simulink library "commblkcod"  (Simulink 5.0)
undefined symbols (not defined in the file or in its folder): G, gfprimfd, H, k, m, n, p
libraries: commutil x28, dspmtrx2 x14, commblkcod x12, commsource x12
settings Model: Creator=mikem  LastModifiedBy=mmclerno

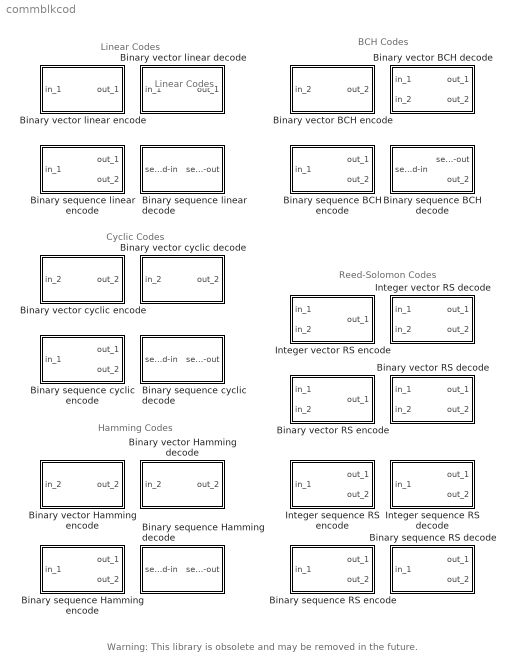
== system commblkcod ==
  note: Linear Codes
  note: Cyclic Codes
  note: Hamming Codes
  note: BCH Codes
  note: Reed-Solomon Codes
  note: Linear Codes
  note: Warning: This library is obsolete and may be removed in the future.
  Binary sequence BCH decode : Subsystem  mask(Sequence I/O BCH decode){n=15, k=5, t=3, samp=1/5}
      mask prompts: n "Codeword length N (N=2^M-1. M is a >2 integer):"; k "Message length K (check BCHPOLY for valid K):"; t "Error-correction capability T (0 for unknown):"; samp "Output sample time T_out (sec):"
      mask help: BCH decode with codeword length N, message length K, and error-correction capability T. (N,K,T) must be a valid BCH code combination.
      mask Help: This block decodes length N binary codeword into length K message using BCH code. The block uses sequential input/output format. The input sequence sample time is K*T_out/N. The block causes a K*T_out delay. The second outport outputs the number of errors detected in the process. A negative value indicates the block found more error in the codeword than T.
      mask Display: plot(0,0,100,100,[35 05 05 35 35 35 15 15 25 25 35 35 60 70 70 75 70 70 75 75 95 95 75 75 85 85],[95 95 85 85 95 85 85 95 95 85 85 90 90 90 93 90 87 93 90 95 95 85 85 95 95 85]-5);disp('BCH de')
  Binary sequence BCH encode : Subsystem  mask(Sequence I/O BCH encode){n=15, k=5, samp=1/5}
      mask prompts: n "Codeword length N (N=2^M-1. M is a >2 integer):"; k "Message length K (check BCHPOLY for valid K):"; samp "Input sample time T_in (sec):"
      mask help: BCH encode with codeword length N, and message length K. (N, K) must be a valid BCH code pair.
      mask init:
      | [x,y]=trigicon(1,75,get_param(gcb,'orientation'),1);
      mask Help: This block encodes length K binary message into length N binary codeword using BCH code. The block uses sequence input/output format. The output sequential sample time is K*T_in/N. The block causes a K*T_in delay. The second outport outputs a pulse when Kth message signal is received. Use function BCHPOLY to view the valid N, K, and error-corr ection capability T combination.
      mask Display: plot(0,0,100,100, [25 5 5 25 25 25 15 15 25 25 50 60 60 65 60 60 65 65 95 95 65 65 75 75 85 85],[90 90 80 80 90 80 80 90 90 85 85 85 88 85 82 88 85 90 90 80 80 90 90 80 80 90],x,y);disp('BCH en')
  Binary sequence Hamming decode : Subsystem  mask(Sequence I/O Hamming decode){n=7, k=gfprimfd(3,'min'), samp=1/4}
      mask prompts: n "Codeword length N:"; k "Message length K, or M-degree primitive polynomial:"; samp "Input sample time T_out (sec):"
      mask help: Single error-correction Hamming decode with codeword length N=2^M-1, message length K=2^M-M-1, where M is a >=3 integer.
      mask init:
      | if length(k)>1,p=k;k=n-length(p)+1;else,p=gfprimdf(n-k);end;
      mask Help: This block decodes length N binary codeword into length K message using Hamming code. The block uses sequential input/output format. The input sequence sample time is K*T_out/N. The block causes a K*T_out delay. Use function GFPRIMDF or GFPRIMFD to find M-degree\nprimitive polynomials.
      mask Display:
      | plot(0,0,100,100,[35 05 05 35 35 35 15 15 25 25 35 35 60 70 70 75 70 70 75 75 95 95 75 75 85 85],[95 95 85 85 95 85 85 95 95 85 85 90 90 90 93 90 87 93 90 95 95 85 85 95 95 85]-5);
      | disp('Hamming de')
  Binary sequence Hamming encode : Subsystem  mask(Sequence I/O Hamming encode){n=7, k=gfprimfd(3,'min'), samp=1/4}
      mask prompts: n "Codeword length N:"; k "Message length K, or M-degree primitive polynomial:"; samp "Input sample time T_in (sec):"
      mask help: Single error-correction Hamming encode with codeword length N=2^M-1, message length K=2^M-M-1, where M is a >=3 integer.
      mask init:
      | if length(k)>1,p=k;k=n-length(k)+1;else,p=gfprimdf(n-k);end;
      mask Help: This block encodes length K binary message into length N binary codeword using Hamming code. The block uses sequential input/output format. The output sequence sample time is K*T_in/N. The block causes a K*T_in delay. The second outport outputs a pulse when Kth message signal is received. Use function GFPRIMDF or GFPRIMFD to find M-degree\nprimitive polynomials.
      mask Display:
      | plot(0,0,100,100, [25 5 5 25 25 25 15 15 25 25 50 60 60 65 60 60 65 65 95 95 65 65 75 75 85 85],[90 90 80 80 90 80 80 90 90 85 85 85 88 85 82 88 85 90 90 80 80 90 90 80 80 90]);
      | disp('Hamming en')
  Binary sequence RS decode : Subsystem  mask(Binary sequence I/O RS decode){n=7, k=5, samp=1/5/3}
      mask prompts: n "Code length N=2^M-1 (M is a >2 integer):"; k "Message length K:"; samp "Output sample time T_out (sec):"
      mask help: RS decode with codeword length N, message length K.
      mask init:
      | m=3;p_d=7;while p_d<n,m=m+1;p_d=2^m-1;end;
      mask Help: This block decodes length N binary codeword into length K binary message. The block uses sequence input/output format. The input sequential sample time is K*T_out/N. The block causes a K*M*T_out delay. The second outport outputs the number of errors detected in the process. If the codeword contains more error than the correction capability, this output is nagative.
      mask Display:
      | plot(0,0,100,100,[35 05 05 35 35 35 15 15 25 25 35 35 60 70 70 75 70 70 75 75 95 95 75 75 85 85],[95 95 85 85 95 85 85 95 95 85 85 90 90 90 93 90 87 93 90 95 95 85 85 95 95 85]-5);
      | disp('B-RS de')
  Binary sequence RS encode : Subsystem  mask(Binary sequence I/O RS encode){n=7, k=5, samp=1/5/3}
      mask prompts: n "Code length N=2^M-1 (M is a >2 integer):"; k "Message length K:"; samp "Input sample time T_in (sec):"
      mask help: RS encode with codeword length N, message length K.
      mask init:
      | m=3;p_m=7;while p_m<n,m=m+1;p_m=2^m-1;end;
      mask Help: This block encodes length K binary message into length N binary codeword. The block uses sequential input/output format. The output sequence sample time is K*T_in/N. The block causes a K*M*T_in delay. The second outport outputs a pulse when (K*M)-th message signal is received.
      mask Display:
      | plot(0,0,100,100, [25 5 5 25 25 25 15 15 25 25 50 60 60 65 60 60 65 65 95 95 65 65 75 75 85 85],[90 90 80 80 90 80 80 90 90 85 85 85 88 85 82 88 85 90 90 80 80 90 90 80 80 90]);
      | disp('B-RS en')
  Binary sequence cyclic decode : Subsystem  mask(Sequence I/O cyclic decode){n=7, p=4, samp=1/4}
      mask prompts: n "Codeword length N:"; p "Message length K, or generator polynomial Pg:"; samp "Output sample time T_out (sec):"
      mask help: Sequence decode with codeword length N and message length K.
      mask init:
      | if length(p)==1, p=cyclpoly(n,p,'min');end;if isempty(p),error('No such cyclic code exist');end;k=n-length(p)+1;
      mask Help: This block decodes length N binary codeword into length K message using cyclic code. The block uses sequential input/output format. Use function CYCLPOLY for a list of cyclic generator polynomials. The input sequence sample time is K*T_out/N. The block causes a K*T_out delay.
      mask Display:
      | plot(0,0,100,100,[35 05 05 35 35 35 15 15 25 25 35 35 60 70 70 75 70 70 75 75 95 95 75 75 85 85],[95 95 85 85 95 85 85 95 95 85 85 90 90 90 93 90 87 93 90 95 95 85 85 95 95 85]-5);
      | disp('Cyclic de');
  Binary sequence cyclic encode : Subsystem  mask(Sequence I/O cyclic encode){n=7, p=4, samp=1/4}
      mask prompts: n "Codeword length N:"; p "Message length K, or generator polynomial Pg:"; samp "Input sample time T_in (sec):"
      mask help: Cyclic encode with codeword length N and message length K.
      mask init:
      | if length(p)==1,p=cyclpoly(n,p,'min');if isempty(p),error('No such cyclic code exist');end;end;k=n-length(p)+1;
      mask Help: This block encodes length K binary message into length N binary codeword using cyclic code. The block uses sequential input/output format. The output sequence sample time is K*T_in/N. The block causes a K*T_in delay. The second outport outputs a pulse when Kth message signal is received. Use function CYCLPOLY for a list of cyclic generator polynomials.
      mask Display:
      | plot(0,0,100,100, [25 5 5 25 25 25 15 15 25 25 50 60 60 65 60 60 65 65 95 95 65 65 75 75 85 85],[90 90 80 80 90 80 80 90 90 85 85 85 88 85 82 88 85 90 90 80 80 90 90 80 80 90]);
      | disp('Cyclic en')
  Binary sequence linear decode : Subsystem  mask(Sequence I/O linear block decode){G=[[1 1 0; 0 1 1; 1 1 1; 1 0 1] eye(4)], trt=0, samp=1/4}
      mask prompts: G "Generator matrix (binary K-by-N matrix):"; trt "Error-correction truth table (0 for single error-corr):"; samp "Output sample time T_out (sec):"
      mask help: Linear block decode with message length K and codeword length N.
      mask init:
      | [k,n]=size(G);
      mask Help: This block decodes length N binary codeword into length K message using linear block code. The block uses sequential input/output format. The input sequence sample time is K*T_out/N. The block causes a K*T_out delay. The generator matrix is a K-by-N matrix. Linear block code is a generic code.
      mask Display:
      | plot(0,0,100,100,[35 05 05 35 35 35 15 15 25 25 35 35 60 70 70 75 70 70 75 75 95 95 75 75 85 85],[95 95 85 85 95 85 85 95 95 85 85 90 90 90 93 90 87 93 90 95 95 85 85 95 95 85]-5);
      | disp('Linear de')
  Binary sequence linear encode : Subsystem  mask(Sequence I/O linear block encode){G=[[1 1 0; 0 1 1; 1 1 1; 1 0 1] eye(4)], samp=1/4}
      mask prompts: G "Generator matrix (binary K-by-N matrix):"; samp "Input sample time T_in (sec):"
      mask help: Linear block encode with message length K and codeword length N.
      mask init:
      | [k, n]=size(G);
      mask Help: This block encodes length K binary message into length N binary codeword using linear block code. The block uses sequential input/output format. The output sequence sample time is K*T_in/N. The block causes a K*T_in delay. The second outport outputs a pulse when Kth message signal is received. The generator matrix is a K-by-N matrix. Linear block code is a generic code.
      mask Display:
      | plot(0,0,100,100, [25 5 5 25 25 25 15 15 25 25 50 60 60 65 60 60 65 65 95 95 65 65 75 75 85 85],[90 90 80 80 90 80 80 90 90 85 85 85 88 85 82 88 85 90 90 80 80 90 90 80 80 90]);
      | disp('Linear en')
  Binary vector BCH decode : Subsystem  mask(Vector I/O BCH decode){n=15, k=5, t=3}
      mask prompts: n "Codeword length N (N=2^M-1. M is a >2 integer):"; k "Message length K (check BCHPOLY for valid K):"; t "Error-correction capability T (0 for unknown):"
      mask help: BCH decode with input codeword vector length N, output message vector length K, and error-correction capability T. (N,K,T) must be a valid BCH code combination.
      mask init:
      | [x,y]=trigicon(0,25,get_param(gcb,'orientation'),1);if t<=0, [x1,x2,x3,x4,t]=bchpoly(n,k);end;dim=3;pow_dim=7;while pow_dim<n,dim=dim+1;pow_dim=2^dim-1;end;tp=gftuple([-1:n-1]',dim);
      mask Help: This block decodes length N binary vector codeword input into length K binary vector message output using BCH code. The block refreshes its decoding output when the enable signal at the second inport has positive value. The second outport outputs the number of errors detected in the process. A negative value indicates the block found more error in the codeword than T.
      mask Display: plot(0,0,100,100,[5 15 15 5 15 15 5 5 15 15 20 15 75 75 85 75 75 15 75 75 85 85 95 95 85 85 95],[75 75 85 85 85 65 65 95 95 83 80 77 77 73 80 87 83 83 83 87 80 90 90 70 70 80 80],x,y);disp('BCH de')
  Binary vector BCH encode : Subsystem  mask(Vector I/O BCH encode){n=15, k=5}
      mask prompts: n "Codeword length N (N=2^M-1. M is a >2 integer):"; k "Message length K (check BCHPOLY for valid K):"
      mask help: BCH encode with input message vector length K and output codeword vector length N. (N, K) must be a valid BCH code pair.
      mask init:
      | pg = bchpoly(n,k);[h,G]=cyclgen(n,pg);
      mask Help: This block encodes length K binary vector message input into length N binary vector codeword output using BCH code. Use function BCHPOLY to view the valid N, K, and error-corr ection capability T combination.
      mask Display: plot(0,0,100,100,[05 15 15 05 05 15 15 15  15 20 15 75 75 85 75 75 15 75 75  85 85 95 95 85 85 95 85 85 95],[80 80 90 90 70 70 90 80  83 80 77 77 73 80 87 83 83 83 87  80 95 95 65 65 85 85 85 75 75]);disp('BCH en')
  Binary vector Hamming decode : Subsystem  mask(Vector I/O Hamming decode){n=7, k=gfprimfd(3,'min')}
      mask prompts: n "Codeword length N:"; k "Message length K, or M-degree primitive polynomial:"
      mask help: Hamming decode with input codeword vector length N=2^M-1, output message vector length K=2^M-M-1, where M is a >=3 integer.
      mask init:
      | if length(k)>1,p=k;k=n-length(p)+1;else,p=gfprimdf(n-k);end;[H,G]=hammgen(n-k,p);trt=htruthtb(G);[n,m]=size(G);G=[zeros(n,m-n),eye(n)];
      mask Help: This block decodes length N binary vector codeword input into length K binary vector message output using Hamming code. Use\nfunction GFPRIMDF or GFPRIMFD to find M-degree primitive polynomials.
      mask Display: plot(0,0,100,100,[1 3 3 1 3 3 1 1 3 3 4 3 15 15 17 15 15 3 15 15 17 17 19 19 17 17 19]*5,[-5 -5 5 5 5 -15 -15 15 15 3 0 -3 -3 -7 0 7 3 3 3 7 0 10 10 -10 -10 0 0]+80);disp('Hamming de')
  Binary vector Hamming encode : Subsystem  mask(Vector I/O Hamming encode){n=7, k=gfprimfd(3,'min')}
      mask prompts: n "Codeword length N:"; k "Message length K, or M-degree primitive polynomial:"
      mask help: Hamming encode with input message vector length K=2^M-M-1, output codeword vector length N=2^M-1, where M is a >=3 integer.
      mask init:
      | if length(k)>1, p=k; k=n-length(k)+1;
      | else, p=gfprimdf(n-k); end;
      | [h,G]=hammgen(n-k,p);
      mask Help: This block encodes length K binary vector message input into length N binary vector codeword output using Hamming code. Use function GFPRIMDF or GFPRIMFD to find M-degree primitive polynomials.
      mask Display: plot(0,0,100,100,[1 3 3 1 1 3 3 3 3 4 3 15 15 17 15 15 3 15 15 17 17 19 19 17 17 19 17 17 19]*5,[0 0 10 10 -10 -10 10 0 3 0 -3 -3 -7 0 7 3 3 3 7 0 15 15 -15 -15 5 5 5 -5 -5]+80);disp('Hamming en')
  Binary vector RS decode : Subsystem  mask(Binary vector I/O RS decode){n=7, k=5}
      mask prompts: n "Code length N=2^M-1 (M is a >2 integer):"; k "Message length K (< N):"
      mask help: Reed-Solomon decode with binary input vector length N*M and binary output vector length K*M.
      mask init:
      | dim=3;p_d=7;while p_d<n,dim=dim+1;p_d=2^dim-1;end;tp=gftuple([-1:n-1]',dim);
      mask Help: This block decodes length N*M binary vector input into length K*M binary vector output. The codeword length is N=2^M-1. M>2. The message length is K<N. The block refreshes its decoding output when the enable signal at the second inport has positive value. The second outport outputs the number of errors detected in the process. If the codeword contains more errors than the correction capability, this output is negative.
      mask Display:
      | plot(0,0,100,100,[5 15 15 5 15 15 5 5 15 15 20 15 75 75 85 75 75 15 75 75 85 85 95 95 85 85 95],[75 75 85 85 85 65 65 95 95 83 80 77 77 73 80 87 83 83 83 87 80 90 90 70 70 80 80],[5 10 10 15 15 20],5*[1 1 2 2 1 1]+10);
      | disp('B-RS de')
  Binary vector RS encode : Subsystem  mask(Binary vector I/O RS encode){n=7, k=5}
      mask prompts: n "Code length N=2^M-1 (M is a >2 integer):"; k "Message length K (< N):"
      mask help: Reed-Solomon encode with binary input vector length K*M and binary output vector length N*M.
      mask init:
      | if length(k)>1,pg=k;k=n-length(pg)-1;else,pg=rspoly(n,k);end;dim=3;p_dim=7;while p_dim<n,dim=dim+1;p_dim=2^dim-1;end;tp=gftuple([-1:n-1]',dim);
      mask Help: This block encodes length K*M binary vector input into length N*M binary vector output. The codeword length is N=2^M-1. M is a integer larger than 2. The message length is K<N. The block refreshes its encoding output when the enable signal at the second inport has positive value.
      mask Display:
      | plot(0,0,100,100,[05 15 15 05 05 15 15 15  15 20 15 75 75 85 75 75 15 75 75  85 85 95 95 85 85 95 85 85 95],[80 80 90 90 70 70 90 80  83 80 77 77 73 80 87 83 83 83 87  80 95 95 65 65 85 85 85 75 75],[5 10 10 15 15 20],5*[1 1 2 2 1 1]+10);
      | disp('B-RS en')
  Binary vector cyclic decode : Subsystem  mask(Vector I/O cyclic decode){n=7, p=4}
      mask prompts: n "Codeword length N:"; p "Message length K, or generator polynomial Pg:"
      mask help: Cyclic decode with codeword length N and message length K.
      mask init:
      | if length(p)==1, p=cyclpoly(n,p,'min');
      |    if isempty(p), error('No cyclic code exists for specified values of Nand K'); end; end;
      | [H,G]=cyclgen(n,p);trt=htruthtb(G);[n,m]=size(G);
      mask Help: This block decodes length N binary vector codeword input into length K binary vector message output using cyclic code. When Pg is specified instead of K, the block uses the user-defined cyclic polynomial Pg. Use function CYCLPOLY for a list of cyclic generator polynomials.
      mask Display:
      | plot(0,0,100,100,[5 15 15 5 15 15 5 5 15 15 20 15 75 75 85 75 75 15 75 75 85 85 95 95 85 85 95],[75 75 85 85 85 65 65 95 95 83 80 77 77 73 80 87 83 83 83 87 80 90 90 70 70 80 80]);
      | disp('Cyclic de')
  Binary vector cyclic encode : Subsystem  mask(Vector I/O cyclic encode){n=7, p=4}
      mask prompts: n "Codeword length N:"; p "Message length K, or generator polynomial Pg:"
      mask help: Cyclic encode with codeword length N and message length K.
      mask init:
      | if length(p)==1,p=cyclpoly(n,p,'min');
      |    if isempty(p),error('No cyclic code exists for specified values of N and K');end;end;
      | [h,G]=cyclgen(n, p);
      mask Help: This block encodes length K binary vector message input into length N binary vector codeword output using cyclic code. When Pg is specified instead of K, the block uses the user-defined cyclic polynomial Pg. Use function CYCLPOLY for a list of cyclic generator polynomials.
      mask Display:
      | plot(0,0,100,100,[05 15 15 05 05 15 15 15  15 20 15 75 75 85 75 75 15 75 75  85 85 95 95 85 85 95 85 85 95],[80 80 90 90 70 70 90 80  83 80 77 77 73 80 87 83 83 83 87  80 95 95 65 65 85 85 85 75 75]);
      | disp('Cyclic en')
  Binary vector linear decode : Subsystem  mask(Vector I/O linear block decode){G=[[1 1 0; 0 1 1; 1 1 1;1 0 1] eye(4)], trt=0}
      mask prompts: G "Generator matrix (binary K-by-N matrix):"; trt "Error-correction truth table (0 for single error-corr):"
      mask help: Linear block decode with input codeword vector length N and output message vector length K.
      mask init:
      | H=gen2par(G);if trt==0,trt=htruthtb(G);end;[n,m]=size(G);
      mask Help: This block decodes length N binary vector codeword input into length K binary vector message output using linear block code. The generator matrix is a K-by-N matrix. Linear block code is a generic code. Use the HTRUTHTB function to generate a single error-correction truth table.
      mask Display:
      | plot(0,0,100,100,[5 15 15 5 15 15 5 5 15 15 20 15 75 75 85 75 75 15 75 75 85 85 95 95 85 85 95],[75 75 85 85 85 65 65 95 95 83 80 77 77 73 80 87 83 83 83 87 80 90 90 70 70 80 80]);
      | disp('Linear de')
  Binary vector linear encode : Subsystem  mask(Vector I/O linear block encode){G=[[1 1 0; 0 1 1; 1 1 1; 1 0 1] eye(4)]}
      mask prompts: G "Generator matrix (binary K-by-N matrix):"
      mask help: Linear block encode with input message vector length K and output codeword vector length N.
      mask Help: Linear block encode with input message vector length K and output codeword vector length N. The generator matrix is a K-by-N matrix. Linear block code is a generic code.
      mask Display:
      | plot(0,0,100,100,[05 15 15 05 05 15 15 15  15 20 15 75 75 85 75 75 15 75 75  85 85 95 95 85 85 95 85 85 95],[80 80 90 90 70 70 90 80  83 80 77 77 73 80 87 83 83 83 87  80 95 95 65 65 85 85 85 75 75]);
      | disp('Linear en')
  Integer sequence RS decode : Subsystem  mask(Integer sequence I/O RS decode){n=7, k=5, samp=1/5}
      mask prompts: n "Code length N=2^M-1 (M is a >2 integer):"; k "Message length K:"; samp "Output sample time T_out (sec):"
      mask help: RS decode with codeword length N, message length K. Input integers are in range [0, N-1].
      mask init:
      | m=3;p_d=7;while p_d<n,m=m+1;p_d=2^m-1;end;
      mask Help: This block decodes length N integer codeword into length K integer message. The block uses sequential input/output format. The input integers are in range [0, N-1]. The input sequence sample time is K*T_out/N. The block causes a K*T_out delay. The second outport outputs the number of errors detected in the process. If the codeword contains more errors than the correction capability, this output is negative.
      mask Display:
      | plot(0,0,100,100,[35 05 05 35 35 35 15 15 25 25 35 35 60 70 70 75 70 70 75 75 95 95 75 75 85 85],[95 95 85 85 95 85 85 95 95 85 85 90 90 90 93 90 87 93 90 95 95 85 85 95 95 85]-5);
      | disp('Int RS de')
  Integer sequence RS encode : Subsystem  mask(Integer sequence I/O RS encode){n=7, k=5, samp=1/5}
      mask prompts: n "Code length N=2^M-1 (M is a >2 integer):"; k "Message length K:"; samp "Input sample time T_in (sec):"
      mask help: RS encode with codeword length N, message length K. Input integers are in range [0, N-1].
      mask init:
      | m=3;p_m=7;while p_m<n,m=m+1;p_m=2^m-1;end;
      mask Help: This block encodes length K integer message into length N integer codeword. The block uses sequential input/output format. The input integers are in range [0, N-1]. The output sequence sample time is K*T_in/N. The block causes a K*T_in delay. The second outport outputs a pulse when Kth message signal is received.
      mask Display:
      | plot(0,0,100,100, [25 5 5 25 25 25 15 15 25 25 50 60 60 65 60 60 65 65 95 95 65 65 75 75 85 85],[90 90 80 80 90 80 80 90 90 85 85 85 88 85 82 88 85 90 90 80 80 90 90 80 80 90]);
      | disp('Int RS en')
  Integer vector RS decode : Subsystem  mask(Integer vector I/O RS decode){n=7, k=5}
      mask prompts: n "Code word length N=2^M-1 (M is a >=3 integer):"; k "Message length K (< N):"
      mask help: Reed-Solomon decode with integer output codeword vector length N and integer input message vector length K.
      mask init:
      | dim=3;p_d=7;while p_d<n,dim=dim+1;p_d=2^dim-1;end;tp=gftuple([-1:n-1]',dim);
      mask Help: This block decodes length N integer vector codeword input into length K integer vector message output. The input/output integers are in the range [0, N-1]. The block refreshes its decoding output when the enable signal at the second inport has positive value. The second outport outputs the number of errors detected in the process. If the codeword contains more errors than the correction capability, this output is negative.
      mask Display:
      | plot(0,0,100,100,[5 15 15 5 15 15 5 5 15 15 20 15 75 75 85 75 75 15 75 75 85 85 95 95 85 85 95],[75 75 85 85 85 65 65 95 95 83 80 77 77 73 80 87 83 83 83 87 80 90 90 70 70 80 80],[5 10 10 15 15 20],5*[1 1 2 2 1 1]+10);
      | disp('Int RS de')
  Integer vector RS encode : Subsystem  mask(Integer vector I/O RS encode){n=7, k=5}
      mask prompts: n "Code length N=2^M-1 (M is a >=3 integer):"; k "Message length K (< N):"
      mask help: Reed-Solomon encode with integer input message vector length K and integer output codeword vector length N.
      mask init:
      | if length(k)>1,pg=k;k=n-length(pg)-1;else,pg=rspoly(n,k);end;dim=3;p_dim=7;while p_dim<n,dim=dim+1;p_dim=2^dim-1;end;tp=gftuple([-1:n-1]',dim);
      mask Help: This block encodes length K integer vector message input into length N integer vector codeword output. The input/output integers are in range [0, N-1]. Code word length N=2^M-1, where M is a integer no less than 3. The message length is K<N. The error-correction capability is T=floor((N-K)/2). The block refreshes its decoding output when the enable signal at the second inport has positive value.
      mask Display:
      | plot(0,0,100,100,[05 15 15 05 05 15 15 15  15 20 15 75 75 85 75 75 15 75 75  85 85 95 95 85 85 95 85 85 95],[80 80 90 90 70 70 90 80  83 80 77 77 73 80 87 83 83 83 87  80 95 95 65 65 85 85 85 75 75],[5 10 10 15 15 20],5*[1 1 2 2 1 1]+10);
      | disp('Int RS en')

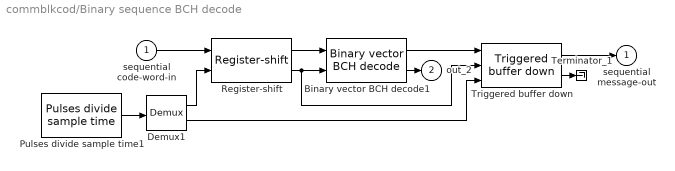
== system commblkcod/Binary sequence BCH decode ==
  sequential code-word-in : Inport
  Binary vector BCH decode1 : commblkcod/Binary vector BCH decode  n=n  k=k  t=t
  Demux1 : Demux  Outputs=2
  Pulses divide sample time1 : commsource/Pulses divide sample time  samp_time=samp*k  out_divid=[n, k]  offset=[0 0]
  Register-shift : commutil/Register-shift  shft_out=[n:-1:1]  thrhld=.1
  Terminator_1 : Terminator
  Triggered buffer down : commutil/Triggered buffer down  in_size=k  ini_idx=0  idx_inc=1  thrshld=.1  cycl_flag=0
  sequential message-out : Outport  InitialOutput=0
  out_2 : Outport  Port=2  InitialOutput=0
  wires:
  Pulses divide sample time1/1 -> Demux1/1
  sequential code-word-in/1 -> Register-shift/1
  Register-shift/1 -> Binary vector BCH decode1/1
  Demux1/1 -> Register-shift/2
  Register-shift/2 -> Triggered buffer down/2, Binary vector BCH decode1/2
  Triggered buffer down/2 -> Terminator_1/1
  Demux1/2 -> Triggered buffer down/3
  Triggered buffer down/1 -> sequential message-out/1
  Binary vector BCH decode1/1 -> Triggered buffer down/1
  Binary vector BCH decode1/2 -> out_2/1

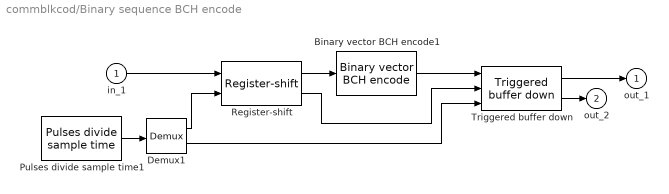
== system commblkcod/Binary sequence BCH encode ==
  in_1 : Inport
  Binary vector BCH encode1 : commblkcod/Binary vector BCH encode  n=n  k=k
  Demux1 : Demux  Outputs=2
  Pulses divide sample time1 : commsource/Pulses divide sample time  samp_time=samp*k  out_divid=[k, n]  offset=[0 0]
  Register-shift : commutil/Register-shift  shft_out=[k:-1:1]  thrhld=.1
  Triggered buffer down : commutil/Triggered buffer down  in_size=n  ini_idx=0  idx_inc=1  thrshld=.1  cycl_flag=0
  out_1 : Outport  InitialOutput=0
  out_2 : Outport  Port=2  InitialOutput=0
  wires:
  Triggered buffer down/2 -> out_2/1
  Triggered buffer down/1 -> out_1/1
  Demux1/2 -> Triggered buffer down/3
  Register-shift/2 -> Triggered buffer down/2
  Binary vector BCH encode1/1 -> Triggered buffer down/1
  Pulses divide sample time1/1 -> Demux1/1
  Demux1/1 -> Register-shift/2
  in_1/1 -> Register-shift/1
  Register-shift/1 -> Binary vector BCH encode1/1

== system commblkcod/Binary sequence Hamming decode ==
  sequential code-word-in : Inport
  Binary vector Hamming decode : commblkcod/Binary vector Hamming decode  n=n  k=p
  Demux : Demux  Outputs=2
  Pulses divide sample time1 : commsource/Pulses divide sample time  samp_time=samp*k  out_divid=[n, k]  offset=[0 0]
  Register-shift : commutil/Register-shift  shft_out=[n:-1:1]  thrhld=.1
  Terminator_1 : Terminator
  Triggered buffer down1 : commutil/Triggered buffer down  in_size=k  ini_idx=0  idx_inc=1  thrshld=.1  cycl_flag=0
  sequential message-out : Outport  InitialOutput=0
  wires:
  Triggered buffer down1/2 -> Terminator_1/1
  Demux/2 -> Triggered buffer down1/3
  Triggered buffer down1/1 -> sequential message-out/1
  Pulses divide sample time1/1 -> Demux/1
  sequential code-word-in/1 -> Register-shift/1
  Binary vector Hamming decode/1 -> Triggered buffer down1/1
  Register-shift/1 -> Binary vector Hamming decode/1
  Register-shift/2 -> Triggered buffer down1/2
  Demux/1 -> Register-shift/2

== system commblkcod/Binary sequence Hamming encode ==
  in_1 : Inport
  Binary vector Hamming encode1 : commblkcod/Binary vector Hamming encode  n=n  k=p
  Demux : Demux  Outputs=2
  Pulses divide sample time1 : commsource/Pulses divide sample time  samp_time=samp*k  out_divid=[k, n]  offset=[0 0]
  Register-shift : commutil/Register-shift  shft_out=[k:-1:1]  thrhld=.1
  Triggered buffer down1 : commutil/Triggered buffer down  in_size=n  ini_idx=0  idx_inc=1  thrshld=.1  cycl_flag=0
  out_1 : Outport  InitialOutput=0
  out_2 : Outport  Port=2  InitialOutput=0
  wires:
  Demux/2 -> Triggered buffer down1/3
  Demux/1 -> Register-shift/2
  Pulses divide sample time1/1 -> Demux/1
  Register-shift/2 -> Triggered buffer down1/2
  in_1/1 -> Register-shift/1
  Register-shift/1 -> Binary vector Hamming encode1/1
  Binary vector Hamming encode1/1 -> Triggered buffer down1/1
  Triggered buffer down1/1 -> out_1/1
  Triggered buffer down1/2 -> out_2/1

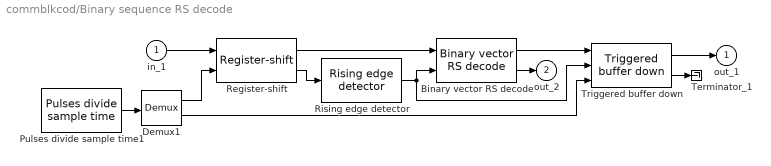
== system commblkcod/Binary sequence RS decode ==
  in_1 : Inport
  Binary vector RS decode : commblkcod/Binary vector RS decode  n=n  k=k
  Demux1 : Demux  Outputs=2
  Pulses divide sample time1 : commsource/Pulses divide sample time  samp_time=samp*k  out_divid=[n, k]  offset=[0 0]
  Register-shift : commutil/Register-shift  shft_out=[n*m:-1:1]  thrhld=.1
  Rising edge detector : commutil/Rising edge detector  thld=0.1
  Terminator_1 : Terminator
  Triggered buffer down : commutil/Triggered buffer down  in_size=k*m  ini_idx=0  idx_inc=1  thrshld=.1  cycl_flag=0
  out_1 : Outport  InitialOutput=0
  out_2 : Outport  Port=2  InitialOutput=0
  wires:
  Triggered buffer down/1 -> out_1/1
  Triggered buffer down/2 -> Terminator_1/1
  Demux1/2 -> Triggered buffer down/3
  Binary vector RS decode/1 -> Triggered buffer down/1
  Register-shift/1 -> Binary vector RS decode/1
  Demux1/1 -> Register-shift/2
  in_1/1 -> Register-shift/1
  Register-shift/2 -> Rising edge detector/1
  Pulses divide sample time1/1 -> Demux1/1
  Binary vector RS decode/2 -> out_2/1
  Rising edge detector/1 -> Triggered buffer down/2, Binary vector RS decode/2

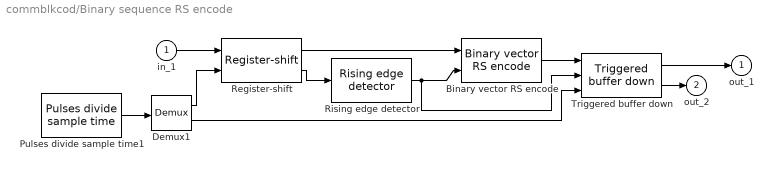
== system commblkcod/Binary sequence RS encode ==
  in_1 : Inport
  Binary vector RS encode : commblkcod/Binary vector RS encode  n=n  k=k
  Demux1 : Demux  Outputs=2
  Pulses divide sample time1 : commsource/Pulses divide sample time  samp_time=samp*k  out_divid=[k, n]  offset=[0 0]
  Register-shift : commutil/Register-shift  shft_out=[k*m:-1:1]  thrhld=.1
  Rising edge detector : commutil/Rising edge detector  thld=0.1
  Triggered buffer down : commutil/Triggered buffer down  in_size=n*m  ini_idx=0  idx_inc=1  thrshld=.1  cycl_flag=0
  out_1 : Outport  InitialOutput=0
  out_2 : Outport  Port=2  InitialOutput=0
  wires:
  Triggered buffer down/1 -> out_1/1
  Triggered buffer down/2 -> out_2/1
  in_1/1 -> Register-shift/1
  Rising edge detector/1 -> Binary vector RS encode/2, Triggered buffer down/2
  Binary vector RS encode/1 -> Triggered buffer down/1
  Demux1/2 -> Triggered buffer down/3
  Register-shift/1 -> Binary vector RS encode/1
  Register-shift/2 -> Rising edge detector/1
  Pulses divide sample time1/1 -> Demux1/1
  Demux1/1 -> Register-shift/2

== system commblkcod/Binary sequence cyclic decode ==
  sequential code-word-in : Inport
  Binary vector cyclic decode : commblkcod/Binary vector cyclic decode  n=n  p=p
  Demux1 : Demux  Outputs=2
  Pulses divide sample time1 : commsource/Pulses divide sample time  samp_time=samp*k  out_divid=[n, k]  offset=[0 0]
  Register-shift : commutil/Register-shift  shft_out=[n:-1:1]  thrhld=.1
  Terminator_1 : Terminator
  Triggered buffer down : commutil/Triggered buffer down  in_size=k  ini_idx=0  idx_inc=1  thrshld=.1  cycl_flag=0
  sequential message-out : Outport  InitialOutput=0
  wires:
  Triggered buffer down/2 -> Terminator_1/1
  Demux1/2 -> Triggered buffer down/3
  Triggered buffer down/1 -> sequential message-out/1
  Pulses divide sample time1/1 -> Demux1/1
  sequential code-word-in/1 -> Register-shift/1
  Binary vector cyclic decode/1 -> Triggered buffer down/1
  Register-shift/1 -> Binary vector cyclic decode/1
  Register-shift/2 -> Triggered buffer down/2
  Demux1/1 -> Register-shift/2

== system commblkcod/Binary sequence cyclic encode ==
  in_1 : Inport
  Binary vector cyclic encode1 : commblkcod/Binary vector cyclic encode  n=n  p=p
  Demux1 : Demux  Outputs=2
  Pulses divide sample time1 : commsource/Pulses divide sample time  samp_time=samp*k  out_divid=[k, n]  offset=[0 0]
  Register-shift : commutil/Register-shift  shft_out=[k:-1:1]  thrhld=.1
  Triggered buffer down : commutil/Triggered buffer down  in_size=n  ini_idx=0  idx_inc=1  thrshld=.1  cycl_flag=0
  out_1 : Outport  InitialOutput=0
  out_2 : Outport  Port=2  InitialOutput=0
  wires:
  Demux1/2 -> Triggered buffer down/3
  Demux1/1 -> Register-shift/2
  Pulses divide sample time1/1 -> Demux1/1
  Register-shift/2 -> Triggered buffer down/2
  Register-shift/1 -> Binary vector cyclic encode1/1
  Binary vector cyclic encode1/1 -> Triggered buffer down/1
  Triggered buffer down/1 -> out_1/1
  Triggered buffer down/2 -> out_2/1
  in_1/1 -> Register-shift/1

== system commblkcod/Binary sequence linear decode ==
  sequential code-word-in : Inport
  Binary vector lin-blk decode1 : commblkcod/Binary vector linear decode  G=G  trt=trt
  Demux1 : Demux  Outputs=2
  Pulses divide sample time1 : commsource/Pulses divide sample time  samp_time=samp*k  out_divid=[n, k]  offset=[0 0]
  Register-shift : commutil/Register-shift  shft_out=[n:-1:1]  thrhld=.1
  Terminator_2 : Terminator
  Triggered buffer down : commutil/Triggered buffer down  in_size=k  ini_idx=0  idx_inc=1  thrshld=.1  cycl_flag=0
  sequential message-out : Outport  InitialOutput=0
  wires:
  Demux1/1 -> Register-shift/2
  Register-shift/2 -> Triggered buffer down/2
  Register-shift/1 -> Binary vector lin-blk decode1/1
  Binary vector lin-blk decode1/1 -> Triggered buffer down/1
  sequential code-word-in/1 -> Register-shift/1
  Pulses divide sample time1/1 -> Demux1/1
  Triggered buffer down/1 -> sequential message-out/1
  Demux1/2 -> Triggered buffer down/3
  Triggered buffer down/2 -> Terminator_2/1

== system commblkcod/Binary sequence linear encode ==
  in_1 : Inport
  Binary vector lin-blk encode1 : commblkcod/Binary vector linear encode  G=G
  Demux1 : Demux  Outputs=2
  Pulses divide sample time1 : commsource/Pulses divide sample time  samp_time=samp*k  out_divid=[k, n]  offset=[0 0]
  Register-shift : commutil/Register-shift  shft_out=[k:-1:1]  thrhld=.1
  Triggered buffer down : commutil/Triggered buffer down  in_size=n  ini_idx=0  idx_inc=1  thrshld=.1  cycl_flag=0
  out_1 : Outport  InitialOutput=0
  out_2 : Outport  Port=2  InitialOutput=0
  wires:
  Triggered buffer down/2 -> out_2/1
  Triggered buffer down/1 -> out_1/1
  Binary vector lin-blk encode1/1 -> Triggered buffer down/1
  Register-shift/1 -> Binary vector lin-blk encode1/1
  in_1/1 -> Register-shift/1
  Register-shift/2 -> Triggered buffer down/2
  Pulses divide sample time1/1 -> Demux1/1
  Demux1/1 -> Register-shift/2
  Demux1/2 -> Triggered buffer down/3

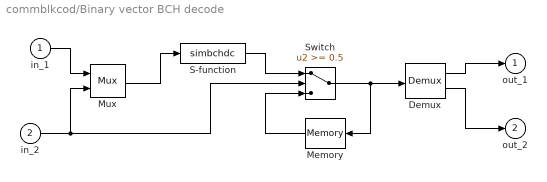
== system commblkcod/Binary vector BCH decode ==
  in_1 : Inport
  in_2 : Inport  Port=2
  Demux : Demux  Outputs=[k, 1]
  Memory : Memory  Orientation=left  X0=zeros(1,k+1)  InheritSampleTime=on
  Mux : Mux  Inputs=[n, 1]
  S-function : S-Function  FunctionName=simbchdc  Parameters=n, k, t,tp,dim
  Switch : Switch  Threshold=0.5  SaturateOnIntegerOverflow=on  InputSameDT=on
  out_1 : Outport  InitialOutput=0
  out_2 : Outport  Port=2  InitialOutput=0
  wires:
  Switch/1 -> Demux/1, Memory/1
  Memory/1 -> Switch/3
  S-function/1 -> Switch/1
  in_1/1 -> Mux/1
  Mux/1 -> S-function/1
  in_2/1 -> Switch/2, Mux/2
  Demux/1 -> out_1/1
  Demux/2 -> out_2/1

== system commblkcod/Binary vector BCH encode ==
  in_2 : Inport
  Constant1 : Constant  Value=2
  Math Function1 : Math  Operator=mod
  Matrix Constant : dspmtrx2/Matrix Constant  M=G
  Matrix Multiplication : dspmtrx2/Matrix Multiplication  Asize=[1 size(G,1)]  Bcols=size(G,2)
  out_2 : Outport  InitialOutput=0
  wires:
  Math Function1/1 -> out_2/1
  Constant1/1 -> Math Function1/2
  Matrix Multiplication/1 -> Math Function1/1
  in_2/1 -> Matrix Multiplication/1
  Matrix Constant/1 -> Matrix Multiplication/2

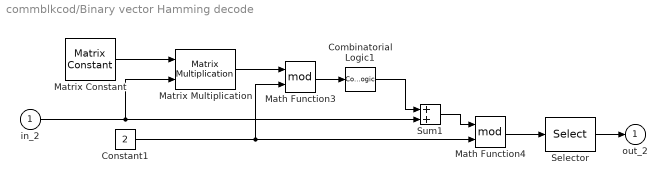
== system commblkcod/Binary vector Hamming decode ==
  in_2 : Inport
  Combinatorial Logic1 : CombinatorialLogic  TruthTable=trt
  Constant1 : Constant  Value=2
  Math Function3 : Math  Operator=mod
  Math Function4 : Math  Operator=mod
  Matrix Constant : dspmtrx2/Matrix Constant  M=H
  Matrix Multiplication : dspmtrx2/Matrix Multiplication  Asize=size(H)  Bcols=1
  Selector : Selector  Elements=[m-n+1:m]  InputPortWidth=m
  Sum1 : Sum  SaturateOnIntegerOverflow=on  InputSameDT=on
  out_2 : Outport  InitialOutput=0
  wires:
  Matrix Multiplication/1 -> Math Function3/1
  Combinatorial Logic1/1 -> Sum1/1
  Sum1/1 -> Math Function4/1
  Math Function4/1 -> Selector/1
  Math Function3/1 -> Combinatorial Logic1/1
  Matrix Constant/1 -> Matrix Multiplication/1
  Selector/1 -> out_2/1
  Constant1/1 -> Math Function3/2, Math Function4/2
  in_2/1 -> Matrix Multiplication/2, Sum1/2

== system commblkcod/Binary vector Hamming encode ==
  in_2 : Inport
  Constant1 : Constant  Value=2
  Math Function1 : Math  Operator=mod
  Matrix Constant : dspmtrx2/Matrix Constant  M=G
  Matrix Multiplication : dspmtrx2/Matrix Multiplication  Asize=[1 size(G,1)]  Bcols=size(G,2)
  out_2 : Outport  InitialOutput=0
  wires:
  Math Function1/1 -> out_2/1
  Constant1/1 -> Math Function1/2
  Matrix Multiplication/1 -> Math Function1/1
  in_2/1 -> Matrix Multiplication/1
  Matrix Constant/1 -> Matrix Multiplication/2

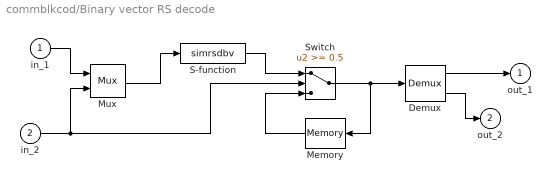
== system commblkcod/Binary vector RS decode ==
  in_1 : Inport
  in_2 : Inport  Port=2
  Demux : Demux  Outputs=[k*dim,1]
  Memory : Memory  Orientation=left  X0=zeros(1,k*dim+1)
  Mux : Mux  Inputs=2
  S-function : S-Function  FunctionName=simrsdbv  Parameters=n, k, tp, dim
  Switch : Switch  Threshold=0.5  SaturateOnIntegerOverflow=on  InputSameDT=on
  out_1 : Outport  InitialOutput=0
  out_2 : Outport  Port=2  InitialOutput=0
  wires:
  Demux/2 -> out_2/1
  Demux/1 -> out_1/1
  in_2/1 -> Mux/2, Switch/2
  Mux/1 -> S-function/1
  in_1/1 -> Mux/1
  S-function/1 -> Switch/1
  Memory/1 -> Switch/3
  Switch/1 -> Memory/1, Demux/1

== system commblkcod/Binary vector RS encode ==
  in_1 : Inport
  in_2 : Inport  Port=2
  Memory : Memory  Orientation=left  X0=zeros(1,n*dim)
  Mux : Mux  Inputs=2
  S-function : S-Function  FunctionName=simrscbv  Parameters=n, k, pg,tp,dim
  Switch : Switch  Threshold=0.5  SaturateOnIntegerOverflow=on  InputSameDT=on
  out_1 : Outport  InitialOutput=0
  wires:
  in_2/1 -> Mux/2, Switch/2
  Mux/1 -> S-function/1
  in_1/1 -> Mux/1
  S-function/1 -> Switch/1
  Memory/1 -> Switch/3
  Switch/1 -> Memory/1, out_1/1

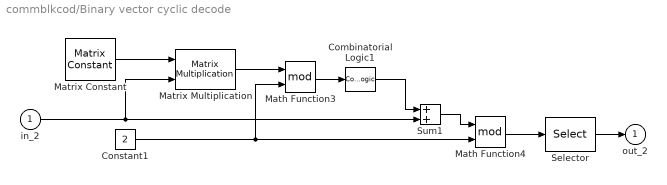
== system commblkcod/Binary vector cyclic decode ==
  in_2 : Inport
  Combinatorial Logic1 : CombinatorialLogic  TruthTable=trt
  Constant1 : Constant  Value=2
  Math Function3 : Math  Operator=mod
  Math Function4 : Math  Operator=mod
  Matrix Constant : dspmtrx2/Matrix Constant  M=H
  Matrix Multiplication : dspmtrx2/Matrix Multiplication  Asize=size(H)  Bcols=1
  Selector : Selector  Elements=[m-n+1:m]  InputPortWidth=m
  Sum1 : Sum  SaturateOnIntegerOverflow=on  InputSameDT=on
  out_2 : Outport  InitialOutput=0
  wires:
  Matrix Multiplication/1 -> Math Function3/1
  Combinatorial Logic1/1 -> Sum1/1
  Sum1/1 -> Math Function4/1
  Math Function4/1 -> Selector/1
  Math Function3/1 -> Combinatorial Logic1/1
  Matrix Constant/1 -> Matrix Multiplication/1
  Selector/1 -> out_2/1
  Constant1/1 -> Math Function4/2, Math Function3/2
  in_2/1 -> Sum1/2, Matrix Multiplication/2

== system commblkcod/Binary vector cyclic encode ==
  in_2 : Inport
  Constant1 : Constant  Value=2
  Math Function1 : Math  Operator=mod
  Matrix Constant : dspmtrx2/Matrix Constant  M=G
  Matrix Multiplication : dspmtrx2/Matrix Multiplication  Asize=[1 size(G,1)]  Bcols=size(G,2)
  out_2 : Outport  InitialOutput=0
  wires:
  Math Function1/1 -> out_2/1
  Constant1/1 -> Math Function1/2
  Matrix Multiplication/1 -> Math Function1/1
  in_2/1 -> Matrix Multiplication/1
  Matrix Constant/1 -> Matrix Multiplication/2

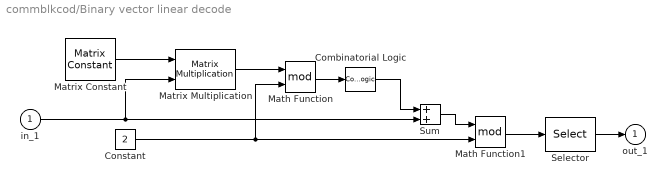
== system commblkcod/Binary vector linear decode ==
  in_1 : Inport
  Combinatorial Logic : CombinatorialLogic  TruthTable=trt
  Constant : Constant  Value=2
  Math Function : Math  Operator=mod
  Math Function1 : Math  Operator=mod
  Matrix Constant : dspmtrx2/Matrix Constant  M=H
  Matrix Multiplication : dspmtrx2/Matrix Multiplication  Asize=size(H)  Bcols=1
  Selector : Selector  Elements=[m-n+1:m]  InputPortWidth=m
  Sum : Sum  SaturateOnIntegerOverflow=on  InputSameDT=on
  out_1 : Outport  InitialOutput=0
  wires:
  Matrix Multiplication/1 -> Math Function/1
  Combinatorial Logic/1 -> Sum/1
  Sum/1 -> Math Function1/1
  Math Function1/1 -> Selector/1
  Math Function/1 -> Combinatorial Logic/1
  Matrix Constant/1 -> Matrix Multiplication/1
  Selector/1 -> out_1/1
  Constant/1 -> Math Function/2, Math Function1/2
  in_1/1 -> Matrix Multiplication/2, Sum/2

== system commblkcod/Binary vector linear encode ==
  in_1 : Inport
  Constant : Constant  Value=2
  Math Function : Math  Operator=mod
  Matrix Constant : dspmtrx2/Matrix Constant  M=G
  Matrix Multiplication : dspmtrx2/Matrix Multiplication  Asize=[1 size(G,1)]  Bcols=size(G,2)
  out_1 : Outport  InitialOutput=0
  wires:
  Math Function/1 -> out_1/1
  Constant/1 -> Math Function/2
  Matrix Multiplication/1 -> Math Function/1
  in_1/1 -> Matrix Multiplication/1
  Matrix Constant/1 -> Matrix Multiplication/2

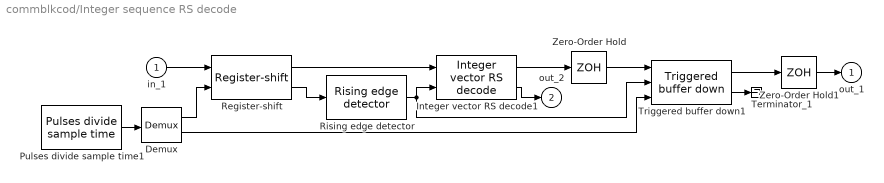
== system commblkcod/Integer sequence RS decode ==
  in_1 : Inport
  Demux : Demux  Outputs=2
  Integer vector RS decode1 : commblkcod/Integer vector RS decode  n=n  k=k
  Pulses divide sample time1 : commsource/Pulses divide sample time  samp_time=samp*k  out_divid=[n, k]  offset=[0 0]
  Register-shift : commutil/Register-shift  shft_out=[n:-1:1]  thrhld=.1
  Rising edge detector : commutil/Rising edge detector  thld=0.1
  Terminator_1 : Terminator
  Triggered buffer down1 : commutil/Triggered buffer down  in_size=k  ini_idx=0  idx_inc=1  thrshld=.1  cycl_flag=0
  Zero-Order Hold : ZeroOrderHold  SampleTime=samp*k
  Zero-Order Hold1 : ZeroOrderHold  SampleTime=samp
  out_1 : Outport  InitialOutput=0
  out_2 : Outport  Port=2  InitialOutput=0
  wires:
  Zero-Order Hold1/1 -> out_1/1
  Triggered buffer down1/1 -> Zero-Order Hold1/1
  Register-shift/1 -> Integer vector RS decode1/1
  Demux/1 -> Register-shift/2
  in_1/1 -> Register-shift/1
  Register-shift/2 -> Rising edge detector/1
  Pulses divide sample time1/1 -> Demux/1
  Triggered buffer down1/2 -> Terminator_1/1
  Integer vector RS decode1/2 -> out_2/1
  Demux/2 -> Triggered buffer down1/3
  Rising edge detector/1 -> Integer vector RS decode1/2, Triggered buffer down1/2
  Integer vector RS decode1/1 -> Zero-Order Hold/1
  Zero-Order Hold/1 -> Triggered buffer down1/1

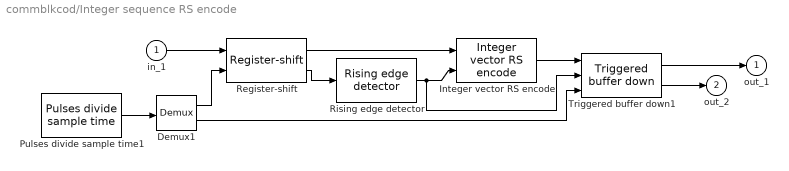
== system commblkcod/Integer sequence RS encode ==
  in_1 : Inport
  Demux1 : Demux  Outputs=2
  Integer vector RS encode : commblkcod/Integer vector RS encode  n=n  k=k
  Pulses divide sample time1 : commsource/Pulses divide sample time  samp_time=samp*k  out_divid=[k, n]  offset=[0 0]
  Register-shift : commutil/Register-shift  shft_out=[k:-1:1]  thrhld=.1
  Rising edge detector : commutil/Rising edge detector  thld=0.1
  Triggered buffer down1 : commutil/Triggered buffer down  in_size=n  ini_idx=0  idx_inc=1  thrshld=.1  cycl_flag=0
  out_1 : Outport  InitialOutput=0
  out_2 : Outport  Port=2  InitialOutput=0
  wires:
  Triggered buffer down1/1 -> out_1/1
  Triggered buffer down1/2 -> out_2/1
  in_1/1 -> Register-shift/1
  Rising edge detector/1 -> Triggered buffer down1/2, Integer vector RS encode/2
  Integer vector RS encode/1 -> Triggered buffer down1/1
  Demux1/2 -> Triggered buffer down1/3
  Register-shift/1 -> Integer vector RS encode/1
  Register-shift/2 -> Rising edge detector/1
  Pulses divide sample time1/1 -> Demux1/1
  Demux1/1 -> Register-shift/2

== system commblkcod/Integer vector RS decode ==
  in_1 : Inport
  in_2 : Inport  Port=2
  Demux : Demux  Outputs=[k, 1]
  Mux : Mux  Inputs=2
  S-function : S-Function  FunctionName=simrsdec  Parameters=n, k, tp, dim
  out_1 : Outport  InitialOutput=0
  out_2 : Outport  Port=2  InitialOutput=0
  wires:
  Demux/2 -> out_2/1
  Demux/1 -> out_1/1
  S-function/1 -> Demux/1
  in_2/1 -> Mux/2
  Mux/1 -> S-function/1
  in_1/1 -> Mux/1

== system commblkcod/Integer vector RS encode ==
  in_1 : Inport
  in_2 : Inport  Port=2
  Mux : Mux  Inputs=2
  S-function : S-Function  FunctionName=simrscod  Parameters=n, k, pg,tp,dim
  out_1 : Outport  InitialOutput=0
  wires:
  S-function/1 -> out_1/1
  in_1/1 -> Mux/1
  Mux/1 -> S-function/1
  in_2/1 -> Mux/2
